simulink model "Ctrls_Software_Strong_Arm_2017b"  (R2017b)
settings: Solver=FixedStepAuto  StartTime=0.0  StopTime=10.0  FixedStep=Ts  RelTol=1e-3  EnableMultiTasking=on
values from neighbouring files (symbols this model uses):
  Ts = .00005    (= 5e-05)    [Setup_Strong_Arm_Parameters.m]
undefined symbols (not defined in the file or in its folder): DiscIntNeverNeededParam, serial
libraries: arduinolib x5, dspsigops x1, instrumentlib x1
settings Model: ExtModeTrigDuration=2  Creator=dtmasetti  LastModifiedBy=Rohan Agarwal
settings OptimizationCC: EnhancedBackFolding=on  PassReuseOutputArgsThreshold=0  MaxStackSize=64  OptimizeBlockOrder=speed  DifferentSizesBufferReuse=on
settings DebuggingCC: ParameterTunabilityLossMsg=error
settings HardwareCC: ProdBitPerInt=16  ProdBitPerPointer=16  ProdBitPerSizeT=16  ProdBitPerPtrDiffT=16  ProdLargestAtomicFloat=None  ProdWordSize=8  ProdHWDeviceType=Atmel->AVR  UseEmbeddedCoderFeatures=off
settings SFSimCC: MATLABDynamicMemAlloc=off
settings RTWCC: SystemTargetFile=ert.tlc  HardwareBoard=Arduino Mega 2560  TLCOptions=-aInlineSetEventsForThisBaseRateFcn=TLC_FALSE -aSuppressMultiTaskScheduler=TLC_FALSE -aRateBasedStepFcn=1  TemplateMakefile=ert_default_tmf  GenerateReport=on  Toolchain=Arduino AVR  BuildConfiguration=Faster Runs  LaunchReport=on
settings CodeAppCC: ForceParamTrailComments=on  OperatorAnnotations=on
settings ERTTargetCC: ERTCustomFileBanners=off  SupportContinuousTime=on  SupportNonInlinedSFcns=on  RemoveResetFunc=off  SupportVariableSizeSignals=on  ModelStepFunctionPrototypeControlCompliant=off

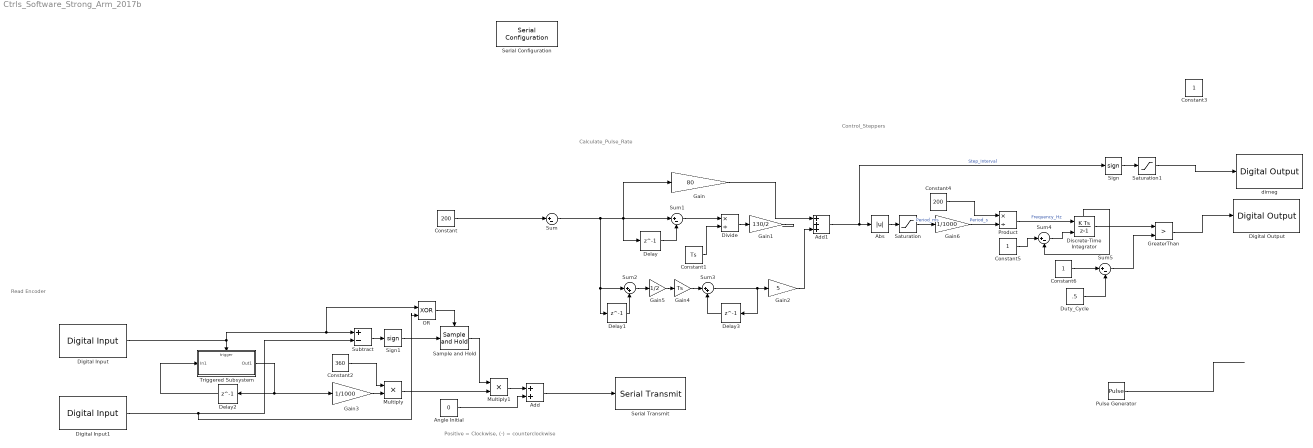
== system Ctrls_Software_Strong_Arm_2017b ==
  note: Calculate_Pulse_Rate
  note: Read Encoder
  note: Control_Steppers
  note: Positive = Clockwise, (-) = counterclockwise
  Abs : Abs
  Add : Sum
  Add1 : Sum  Inputs=+++
  Angle Initial : Constant  Value=0
  Constant : Constant  Value=200
  Constant1 : Constant  Value=Ts
  Constant2 : Constant  Value=360
  Constant3 : Constant
  Constant4 : Constant  Value=200
  Constant5 : Constant
  Constant6 : Constant
  Delay{,1..3} (4 alike) : Delay  DelayLength=1
  Digital Input : arduinolib/Digital Input  pinNumber=18  sampleTime=Ts  blockPlatform=arduino
      settings: SourceProductName=Simulink Support Package for Arduino Hardware
  Digital Input1 : arduinolib/Digital Input  pinNumber=19  sampleTime=Ts  blockPlatform=arduino
      settings: SourceProductName=Simulink Support Package for Arduino Hardware
  Digital Output : arduinolib/Digital Output  pinNumber=26  blockPlatform=arduino
  Discrete-Time Integrator : DiscreteIntegrator  ExternalReset=falling  SampleTime=-1  ShowStatePort=on  ICPrevOutput=DiscIntNeverNeededParam  ICPrevScaledInput=DiscIntNeverNeededParam
  Divide : Product  Inputs=*/
  Duty_Cycle : Constant  Value=.5
  Gain : Gain  Gain=80
  Gain1 : Gain  Gain=130/2
  Gain2 : Gain  Gain=5
  Gain3 : Gain  Gain=1/1000
  Gain4 : Gain  Gain=Ts
  Gain5 : Gain  Gain=1/2
  Gain6 : Gain  Gain=1/1000
  GreaterThan : RelationalOperator  Operator=>  OutDataTypeStr=boolean  RndMeth=Simplest
  Multiply : Product
  Multiply1 : Product
  OR : Logic  Operator=XOR  IconShape=distinctive  AllPortsSameDT=off  OutDataTypeStr=boolean
  Product : Product  Inputs=*/
  Pulse Generator : DiscretePulseGenerator  PulseType=Time based  Period=.001  PulseWidth=50
  Sample and Hold : dspsigops/Sample and Hold  trig=Rising edge  initCond=0  latchinput=off
  Saturation : Saturate  UpperLimit=1000  LowerLimit=300
  Saturation1 : Saturate  UpperLimit=1  LowerLimit=0
  Serial Configuration : instrumentlib/Serial Configuration  Priority=-200000  ComPortMenu=COM10  ComPort=COM10  ObjConstructor=serial('COM10');  BaudRate=9600  DataBits=8  Parity=none  StopBits=1  FlowControl=none  Timeout=10  ByteOrder=LittleEndian
  Serial Transmit : arduinolib/Serial Transmit  portNumber=0  sendmode=println  label=encoder output  sendformat=Decimal  floatprecision=2  blockPlatform=arduino
      settings: SourceProductName=Simulink Support Package for Arduino Hardware
  Sign : Signum
  Sign1 : Signum
  Subtract : Sum  Inputs=+-
  Sum{,1,4..5} (4 alike) : Sum  Inputs=|+-
  Sum2 : Sum  Inputs=|++
  Sum3 : Sum  Inputs=|++
  Triggered Subsystem : Subsystem  TreatAsAtomicUnit=on
  dirneg : arduinolib/Digital Output  pinNumber=24  blockPlatform=arduino
  wires:
  Gain/1 -> Add1/1
  Delay/1 -> Sum1/2
  Sum1/1 -> Divide/1
  Constant1/1 -> Divide/2
  Divide/1 -> Gain1/1
  Gain1/1 -> ?
  Delay1/1 -> Sum2/2
  Gain2/1 -> Add1/3
  Add1/1 -> Abs/1, Sign/1  "Step_Interval"
  Saturation/1 -> Gain6/1  "Period_ms"
  Sign/1 -> Saturation1/1
  Saturation1/1 -> dirneg/1
  Angle Initial/1 -> Add/2
  Constant2/1 -> Multiply/1
  Gain3/1 -> Multiply/2
  Multiply/1 -> Multiply1/2
  Add/1 -> Serial Transmit/1
  Digital Input/1 -> OR/1, Subtract/1, Triggered Subsystem/Trigger
  Digital Input1/1 -> Subtract/2, OR/2
  Triggered Subsystem/1(Out1) -> Gain3/1, Delay2/1
  Delay2/1 -> Triggered Subsystem/1(In1)
  Subtract/1 -> Sign1/1
  Sign1/1 -> Sample and Hold/1
  OR/1 -> Sample and Hold/Trigger
  Sample and Hold/1 -> Multiply1/1
  Multiply1/1 -> Add/1
  Sum2/1 -> Gain5/1
  Sum/1 -> Sum2/1, Delay1/1, Sum1/1, Delay/1, Gain/1
  Gain4/1 -> Sum3/1
  Gain5/1 -> Gain4/1
  Sum3/1 -> Delay3/1, Gain2/1
  Delay3/1 -> Sum3/2
  Constant4/1 -> Product/1
  Product/1 -> Discrete-Time Integrator/1  "Frequency_Hz"
  Gain6/1 -> Product/2  "Period_s"
  Discrete-Time Integrator/1 -> GreaterThan/1
  Constant5/1 -> Sum4/1
  Sum4/1 -> Discrete-Time Integrator/2
  Duty_Cycle/1 -> Sum5/2
  Constant6/1 -> Sum5/1
  Sum5/1 -> GreaterThan/2
  GreaterThan/1 -> Digital Output/1
  Discrete-Time Integrator/State -> Sum4/2
  Pulse Generator/1 -> ?
  Constant/1 -> Sum/1
  Abs/1 -> Saturation/1

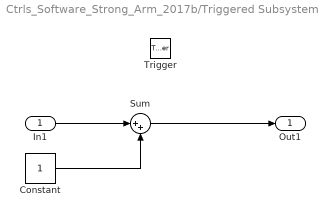
== system Ctrls_Software_Strong_Arm_2017b/Triggered Subsystem ==
  In1 : Inport
  Trigger : TriggerPort  VariantControl=Variant
  Constant : Constant
  Sum : Sum  Inputs=|++
  Out1 : Outport
  wires:
  In1/1 -> Sum/1
  Constant/1 -> Sum/2
  Sum/1 -> Out1/1
